simulink model "zadanie"  (R2018b)
settings: Solver=VariableStepAuto  StartTime=0.0  StopTime=10.0  RelTol=1e-3
settings Model: Creator=michask  LastModifiedBy=michask

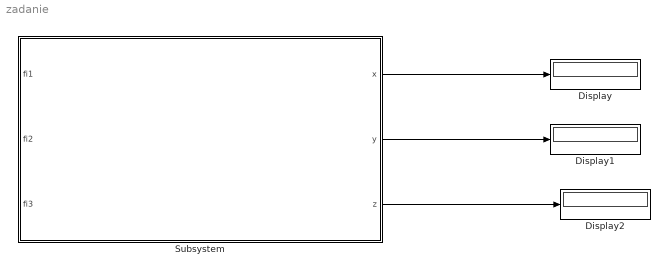
== system zadanie ==
  Display : Display
  Display1 : Display
  Display2 : Display
  Subsystem : Subsystem
  wires:
  Subsystem/1(x) -> Display/1
  Subsystem/2(y) -> Display1/1
  Subsystem/3(z) -> Display2/1

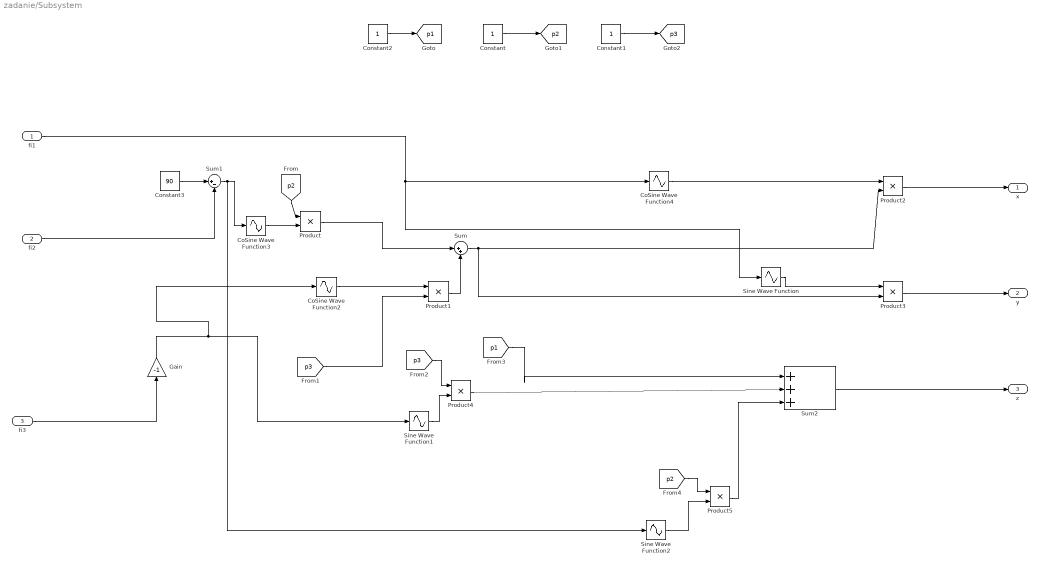
== system zadanie/Subsystem ==
  fi1 : Inport
  fi2 : Inport  Port=2
  fi3 : Inport  Port=3
  CoSine Wave Function2 : Sin  TimeSource=Use external signal  Phase=1.57079  SampleTime=0
  CoSine Wave Function3 : Sin  TimeSource=Use external signal  Phase=1.57079  SampleTime=0
  CoSine Wave Function4 : Sin  TimeSource=Use external signal  Phase=1.57079  SampleTime=0
  Constant : Constant
  Constant1 : Constant
  Constant2 : Constant
  Constant3 : Constant  Value=90
  Gain : Gain  Gain=-1
  Product{,1..5} (6 alike) : Product
  Sine Wave Function : Sin  TimeSource=Use external signal  SampleTime=0
  Sine Wave Function1 : Sin  TimeSource=Use external signal  SampleTime=0
  Sine Wave Function2 : Sin  TimeSource=Use external signal  SampleTime=0
  Sum : Sum  Inputs=|++
  Sum1 : Sum  Inputs=|+-
  Sum2 : Sum  Inputs=|+++
  x : Outport
  y : Outport  Port=2
  z : Outport  Port=3
  tag scope: p1=global, p2=global, p3=global
  wires:
  CoSine Wave Function4/1 -> Product2/1
  fi1/1 -> Sine Wave Function/1, CoSine Wave Function4/1
  Constant2/1 -> [p1]
  Constant/1 -> [p2]
  Constant1/1 -> [p3]
  Sum/1 -> Product3/2, Product2/2
  Product2/1 -> x/1
  [p3] -> Product1/2
  fi3/1 -> Gain/1
  Gain/1 -> Sine Wave Function1/1, CoSine Wave Function2/1
  CoSine Wave Function2/1 -> Product1/1
  [p2] -> Product/1
  Constant3/1 -> Sum1/1
  fi2/1 -> Sum1/2
  Product/1 -> Sum/1
  Product1/1 -> Sum/2
  CoSine Wave Function3/1 -> Product/2
  Sine Wave Function/1 -> Product3/1
  Product3/1 -> y/1
  [p3] -> Product4/1
  Sine Wave Function1/1 -> Product4/2
  Product4/1 -> Sum2/2
  [p1] -> Sum2/1
  [p2] -> Product5/1
  Sum1/1 -> Sine Wave Function2/1, CoSine Wave Function3/1
  Sum2/1 -> z/1
  Product5/1 -> Sum2/3
  Sine Wave Function2/1 -> Product5/2
